simulink model "PID_controller_lat"  (R2019a)
settings: Solver=VariableStepAuto  StartTime=0.0  StopTime=50  FixedStep=1e-5  RelTol=1e-3
values from neighbouring files (symbols this model uses):
  sys = ss(A,B,C,D,'StateName', {'u'; 'w'; 'q'; 'theta'; 'h'}, 'InputName', {'eta';'epsilon'})    [control_system_v01.m]    (also in control_system_v02.m = ss(A,B,C,D,'StateName', {'u'; 'w'; 'q'; 'theta'},          ')
undefined symbols (not defined in the file or in its folder): a, b, c, env, F, Light, MIL
libraries: aerolibactuator x2, simulink x2, hdlsllib x1, aerolibwind2 x1, dspmtrx3 x1
settings Model: Creator=tyson  LastModifiedBy=tyson
settings DebuggingCC: InheritedTsInSrcMsg=none

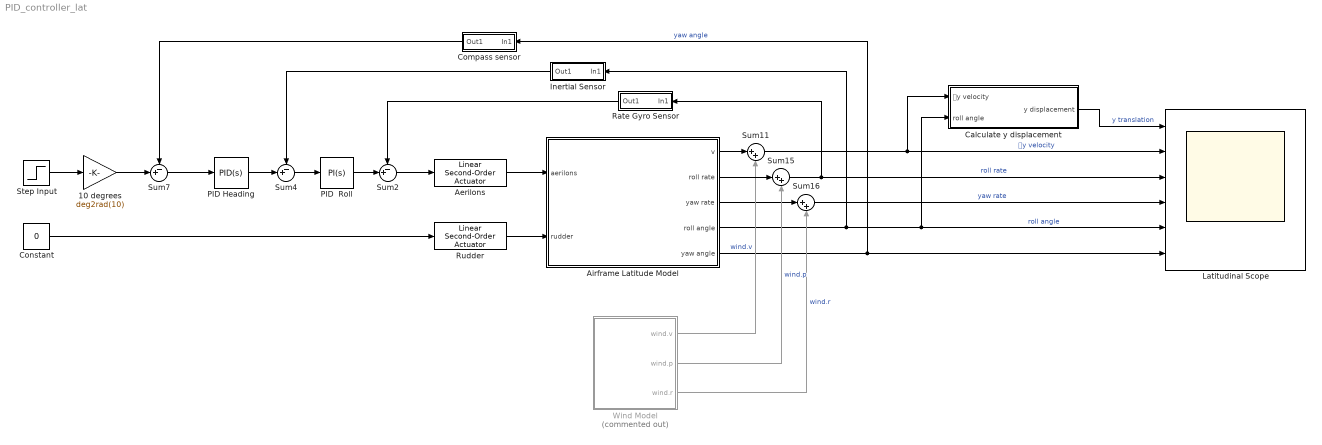
== system PID_controller_lat ==
  10 degrees : Gain  Gain=deg2rad(10)
  Aerilons : aerolibactuator/Linear Second-Order Actuator  wn_fin=actuators.naturalFreq  z_fin=actuators.dampingRatio  fin_act_0=0  fin_act_vel=0
      settings: SourceProductName=Aerospace Blockset  SourceProductBaseCode=AE
  Airframe Latitude Model : Subsystem
      mask Display: image('/home/tyson/Dropbox/Academic/4th Year/ELEN4011/matlab/icons/airframe_lat.png');
  Calculate y displacement : Subsystem
  Compass sensor : Subsystem
  Constant : Constant  Value=0
  Inertial Sensor : Subsystem
  Latitudinal Scope : Scope  NumInputPorts=6
  PID  Roll : simulink/Continuous/PID Controller  Controller=PI  Form=Parallel  TimeDomain=Continuous-time  SampleTime=-1  IntegratorMethod=Forward Euler  FilterMethod=Forward Euler  ControllerParametersSource=internal  P=13.8346091340675  I=2.4410545354894  D=0  UseFilter=on  N=100  TunerSelectOption=Transfer Function Based (PID Tuner App)  InitialConditionSource=internal  InitialConditionForIntegrator=0  InitialConditionForFilter=0  DifferentiatorICPrevScaledInput=0  ExternalReset=none  TrackingMode=off  Kt=1  LimitOutput=off  UpperSaturationLimit=inf  LowerSaturationLimit=-inf  LinearizeAsGain=on  AntiWindupMode=none  Kb=1  POutMin=[]  POutMax=[]  IOutMin=[]  IOutMax=[]  DOutMin=[]  DOutMax=[]  NOutMin=[]  NOutMax=[]  SumOutMin=[]  SumOutMax=[]  SaturationOutMin=[]  SaturationOutMax=[]  PParamMin=[]  PParamMax=[]  IParamMin=[]  IParamMax=[]  DParamMin=[]  DParamMax=[]  NParamMin=[]  NParamMax=[]  KbParamMin=[]  KbParamMax=[]  KtParamMin=[]  KtParamMax=[]  KbOutMin=[]  KbOutMax=[]  KtOutMin=[]  KtOutMax=[]  IntegratorOutMin=[]  IntegratorOutMax=[]  FilterOutMin=[]  FilterOutMax=[]  SumI1OutMin=[]  SumI1OutMax=[]  SumI2OutMin=[]  SumI2OutMax=[]  SumI3OutMin=[]  SumI3OutMax=[]  SumI4OutMin=[]  SumI4OutMax=[]  SumDOutMin=[]  SumDOutMax=[]  DifferentiatorOutMin=[]  DifferentiatorOutMax=[]  FilterDiffOutCoefMin=[]  FilterDiffOutCoefMax=[]  ReciprocalOutMin=[]  ReciprocalOutMax=[]  SumDenOutMin=[]  SumDenOutMax=[]  SumNumOutMin=[]  SumNumOutMax=[]  DivideOutMin=[]  DivideOutMax=[]  IntegratorContinuousStateAttributes=''  IntegratorStateMustResolveToSignalObject=off  IntegratorRTWStateStorageClass=Auto  FilterContinuousStateAttributes=''  FilterStateMustResolveToSignalObject=off  FilterRTWStateStorageClass=Auto  ParallelPVariant=InternalParameters  IdealPVariant=Disabled  IVariant=InternalParameters  DVariant=Disabled  IntegratorVariant=Continuous  SatVariant=Disabled  AWVariant=Passthrough  PCopyVariant=Disabled  TRVariant=Disabled  FdbkBlocksVariant=Forward  IdealPFdbkVariant=Disabled  SatFdbkVariant=Disabled  DerivativeFilterVariant=Disabled  NVariant=Disabled  NCopyVariant=Disabled_SignalSpec  FilterICVariant=Disabled  IntegratorICVariant=InternalICs  ExternalResetVariant=Disabled  TRSumVariant=Passthrough  SumFdbkVariant=Disabled  SumVariant=Sum_PI
  PID Heading : simulink/Continuous/PID Controller  Controller=PID  Form=Parallel  TimeDomain=Continuous-time  SampleTime=-1  IntegratorMethod=Forward Euler  FilterMethod=Forward Euler  ControllerParametersSource=internal  P=1.21069845200907  I=0.0055970895188787  D=0.229410917426781  UseFilter=on  N=5.54692256878503  TunerSelectOption=Transfer Function Based (PID Tuner App)  InitialConditionSource=internal  InitialConditionForIntegrator=0  InitialConditionForFilter=0  DifferentiatorICPrevScaledInput=0  ExternalReset=none  TrackingMode=off  Kt=1  LimitOutput=off  UpperSaturationLimit=inf  LowerSaturationLimit=-inf  LinearizeAsGain=on  AntiWindupMode=none  Kb=1  POutMin=[]  POutMax=[]  IOutMin=[]  IOutMax=[]  DOutMin=[]  DOutMax=[]  NOutMin=[]  NOutMax=[]  SumOutMin=[]  SumOutMax=[]  SaturationOutMin=[]  SaturationOutMax=[]  PParamMin=[]  PParamMax=[]  IParamMin=[]  IParamMax=[]  DParamMin=[]  DParamMax=[]  NParamMin=[]  NParamMax=[]  KbParamMin=[]  KbParamMax=[]  KtParamMin=[]  KtParamMax=[]  KbOutMin=[]  KbOutMax=[]  KtOutMin=[]  KtOutMax=[]  IntegratorOutMin=[]  IntegratorOutMax=[]  FilterOutMin=[]  FilterOutMax=[]  SumI1OutMin=[]  SumI1OutMax=[]  SumI2OutMin=[]  SumI2OutMax=[]  SumI3OutMin=[]  SumI3OutMax=[]  SumI4OutMin=[]  SumI4OutMax=[]  SumDOutMin=[]  SumDOutMax=[]  DifferentiatorOutMin=[]  DifferentiatorOutMax=[]  FilterDiffOutCoefMin=[]  FilterDiffOutCoefMax=[]  ReciprocalOutMin=[]  ReciprocalOutMax=[]  SumDenOutMin=[]  SumDenOutMax=[]  SumNumOutMin=[]  SumNumOutMax=[]  DivideOutMin=[]  DivideOutMax=[]  IntegratorContinuousStateAttributes=''  IntegratorStateMustResolveToSignalObject=off  IntegratorRTWStateStorageClass=Auto  FilterContinuousStateAttributes=''  FilterStateMustResolveToSignalObject=off  FilterRTWStateStorageClass=Auto  ParallelPVariant=InternalParameters  IdealPVariant=Disabled  IVariant=InternalParameters  DVariant=InternalParameters  IntegratorVariant=Continuous  SatVariant=Disabled  AWVariant=Passthrough  PCopyVariant=Disabled  TRVariant=Disabled  FdbkBlocksVariant=Forward  IdealPFdbkVariant=Disabled  SatFdbkVariant=Disabled  DerivativeFilterVariant=ContFilter  NVariant=InternalParameters  NCopyVariant=Disabled  FilterICVariant=InternalICsFilter  IntegratorICVariant=InternalICs  ExternalResetVariant=Disabled  TRSumVariant=Passthrough  SumFdbkVariant=Disabled  SumVariant=Sum_PID
  Rate Gyro Sensor : Subsystem
  Rudder : aerolibactuator/Linear Second-Order Actuator  wn_fin=actuators.naturalFreq  z_fin=actuators.dampingRatio  fin_act_0=0  fin_act_vel=0
      settings: SourceProductName=Aerospace Blockset  SourceProductBaseCode=AE
  Step Input : Step  Time=0
  Sum11 : Sum  Inputs=|++
  Sum15 : Sum  Inputs=|++
  Sum16 : Sum  Inputs=|++
  Sum2 : Sum  Inputs=-+|
  Sum4 : Sum  Inputs=-+|
  Sum7 : Sum  Inputs=-+|
  Wind Model : Subsystem  Commented=on
      mask Display: image('/home/tyson/Dropbox/Academic/4th Year/ELEN4011/matlab/icons/wind.png');
  wires:
  Step Input/1 -> 10 degrees/1
  Airframe Latitude Model/5(yaw angle) -> Latitudinal Scope/6, Compass sensor/1(In1)  "yaw angle"
  Calculate y displacement/1(y displacement) -> Latitudinal Scope/1  "y translation"
  Airframe Latitude Model/3(yaw rate) -> Sum16/1
  Sum7/1 -> PID Heading/1
  Sum16/1 -> Latitudinal Scope/4  "yaw rate"
  10 degrees/1 -> Sum7/2
  Sum11/1 -> Calculate y displacement/1(𝚫y velocity), Latitudinal Scope/2  "𝚫y velocity"
  Sum15/1 -> Latitudinal Scope/3, Rate Gyro Sensor/1(In1)  "roll rate"
  Aerilons/1 -> Airframe Latitude Model/1(aerilons)
  Airframe Latitude Model/1(v) -> Sum11/1
  Airframe Latitude Model/4(roll angle) -> Latitudinal Scope/5, Calculate y displacement/2(roll angle), Inertial Sensor/1(In1)  "roll angle"
  Sum2/1 -> Aerilons/1
  PID  Roll/1 -> Sum2/2
  Wind Model/1(wind.v) -> Sum11/2  "wind.v"
  Wind Model/2(wind.p) -> Sum15/2  "wind.p"
  Wind Model/3(wind.r) -> Sum16/2  "wind.r"
  Sum4/1 -> PID  Roll/1
  Rate Gyro Sensor/1(Out1) -> Sum2/1
  Inertial Sensor/1(Out1) -> Sum4/1
  Compass sensor/1(Out1) -> Sum7/1
  Constant/1 -> Rudder/1
  Airframe Latitude Model/2(roll rate) -> Sum15/1
  PID Heading/1 -> Sum4/2
  Rudder/1 -> Airframe Latitude Model/2(rudder)

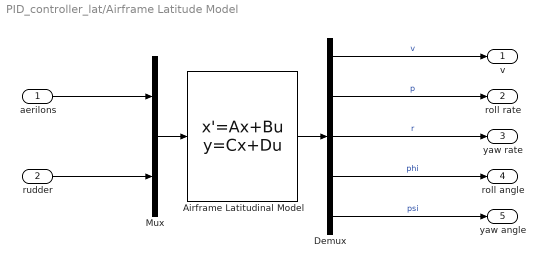
== system PID_controller_lat/Airframe Latitude Model ==
  aerilons : Inport
  rudder : Inport  Port=2
  Airframe Latitudinal Model : StateSpace  A=sys.lat.A  B=sys.lat.B  C=sys.lat.C  D=sys.lat.D  InitialCondition=0
  Demux : Demux  Outputs=5
  Mux : Mux  Inputs=2
  v : Outport
  roll rate : Outport  Port=2
  yaw rate : Outport  Port=3
  roll angle : Outport  Port=4
  yaw angle : Outport  Port=5
  wires:
  rudder/1 -> Mux/2
  Demux/4 -> roll angle/1  "phi"
  Demux/3 -> yaw rate/1  "r"
  Mux/1 -> Airframe Latitudinal Model/1
  Airframe Latitudinal Model/1 -> Demux/1
  Demux/1 -> v/1  "v"
  Demux/2 -> roll rate/1  "p"
  Demux/5 -> yaw angle/1  "psi"
  aerilons/1 -> Mux/1

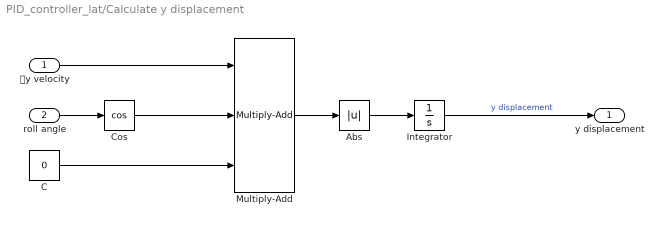
== system PID_controller_lat/Calculate y displacement ==
  𝚫y velocity : Inport
  roll angle : Inport  Port=2
  Abs : Abs
  C : Constant  Value=0
  Cos : Trigonometry  Operator=cos
  Integrator : Integrator
  Multiply-Add : hdlsllib/HDL Operations/Multiply-Add  Function=c+(a.*b)  datatype=Inherit: Inherit via internal rule  DoSatur=off  FMA=off
      settings: SourceProductName=Simulink  SourceProductBaseCode=SL
  y displacement : Outport
  wires:
  C/1 -> Multiply-Add/3
  Abs/1 -> Integrator/1
  Cos/1 -> Multiply-Add/2
  roll angle/1 -> Cos/1
  Integrator/1 -> y displacement/1  "y displacement"
  𝚫y velocity/1 -> Multiply-Add/1
  Multiply-Add/1 -> Abs/1

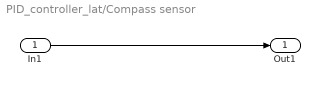
== system PID_controller_lat/Compass sensor ==
  In1 : Inport
  Out1 : Outport
  wires:
  In1/1 -> Out1/1

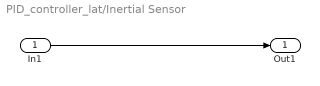
== system PID_controller_lat/Inertial Sensor ==
  In1 : Inport
  Out1 : Outport
  wires:
  In1/1 -> Out1/1

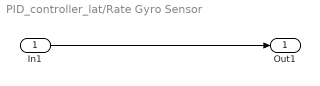
== system PID_controller_lat/Rate Gyro Sensor ==
  In1 : Inport
  Out1 : Outport
  wires:
  In1/1 -> Out1/1

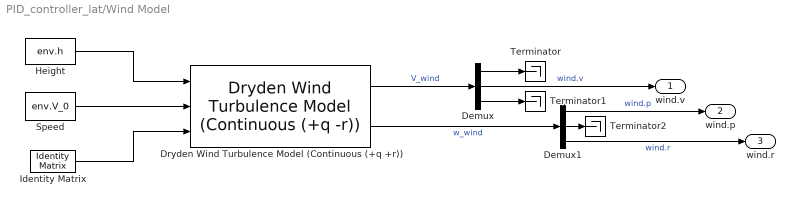
== system PID_controller_lat/Wind Model ==
  Demux : Demux  Outputs=3
  Demux1 : Demux  Outputs=3
  Dryden Wind Turbulence Model (Continuous (+q +r)) : aerolibwind2/Dryden Wind Turbulence Model  (Continuous (+q -r))  units=Metric (MKS)  spec=MIL-F-8785C  model=Continuous Dryden (+q +r)  W20=10  Wdeg=0  TurbProb=10^-2 - Light  L_high=533.4  Wingspan=geometry.b  ts=0.1  Seed=[2541 2542 2543 2544]  T_on=on
      settings: SourceProductName=Aerospace Blockset
  Height : Constant  Value=env.h
  Identity Matrix : dspmtrx3/Identity Matrix  Inherit=off  N=3  Ts=1  dataType=double  isSigned=on  wordLen=16  udDataType=sfix(16)  fracBitsMode=Best precision  numFracBits=15  OutDataTypeStr=double  LastOutDataTypeStr=double
      settings: SourceProductName=DSP System Toolbox
  Speed : Constant  Value=env.V_0
  Terminator : Terminator
  Terminator1 : Terminator
  Terminator2 : Terminator
  wind.v : Outport
  wind.p : Outport  Port=2
  wind.r : Outport  Port=3
  wires:
  Demux/2 -> wind.v/1  "wind.v"
  Demux/3 -> Terminator1/1
  Demux1/3 -> wind.r/1  "wind.r"
  Demux1/2 -> Terminator2/1
  Demux/1 -> Terminator/1
  Dryden Wind Turbulence Model (Continuous (+q +r))/2 -> Demux1/1  "w_wind"
  Demux1/1 -> wind.p/1  "wind.p"
  Height/1 -> Dryden Wind Turbulence Model (Continuous (+q +r))/1
  Dryden Wind Turbulence Model (Continuous (+q +r))/1 -> Demux/1  "V_wind"
  Speed/1 -> Dryden Wind Turbulence Model (Continuous (+q +r))/2
  Identity Matrix/1 -> Dryden Wind Turbulence Model (Continuous (+q +r))/3
